simulink model "dom_TExt"  (R2024a)
settings: Solver=ode45  StartTime=0  StopTime=86400  MaxStep=tMaxStep  RelTol=1e-3
values from neighbouring files (symbols this model uses):
  tSecDay = 24*60*60    (= 86400)    [dom_ogrzewanie_par.m]
  tSecYear = 52*tSecWeek    (= 31449600)    [dom_ogrzewanie_par.m]
settings Model: LastModifiedBy=Kamil Kowalczyk

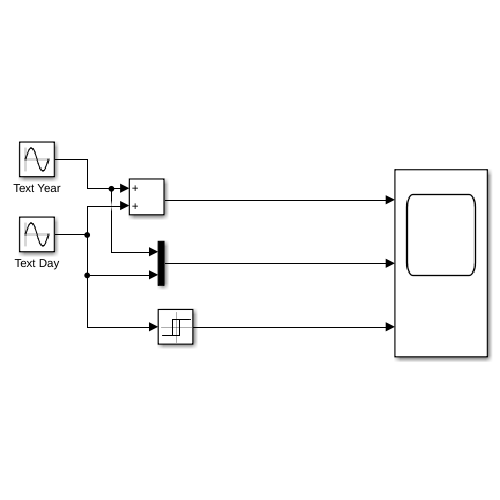
[thumbnail: Simulink's stored preview of the top-level diagram]
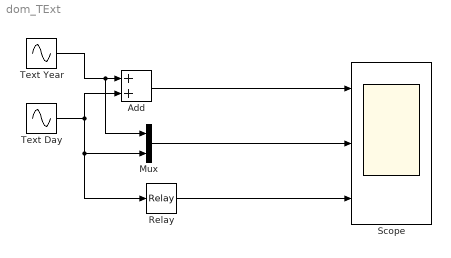
== system dom_TExt ==
  Add : Sum
  Mux : Mux  Inputs=2
  Relay : Relay  OnSwitchValue=1  OffSwitchValue=-0.5
  Scope : Scope  NumInputPorts=3
  Text Day : Sin  Amplitude=5  Frequency=2*pi/tSecDay  SampleTime=0
  Text Year : Sin  Amplitude=15  Bias=10  Frequency=2*pi/tSecYear  SampleTime=0
  wires:
  Text Year/1 -> Mux/1, Add/1
  Text Day/1 -> Relay/1, Mux/2, Add/2
  Add/1 -> Scope/1
  Mux/1 -> Scope/2
  Relay/1 -> Scope/3
